simulink model "regulator_linear_2oder_T2"  (R2022b)
settings: Solver=VariableStepAuto  StartTime=0.0  StopTime=5  FixedStep=0.000001  RelTol=1e-3
values from neighbouring files (symbols this model uses):
  A = [0 1; -a0 -a1]    [analysis_effect_T.m]    (also in regulation_paramters.m)
  B = [b1; b0]    [analysis_effect_T.m]    (also in regulation_paramters.m)
  Pa = Popt    [analysis_effect_T.m]    (also in regulation_paramters.m)
  Q = eye(2)    [analysis_effect_T.m]    (also in regulation_paramters.m)
  R = 1    [analysis_effect_T.m]    (also in regulation_paramters.m)
  T2 = 0.005    [analysis_effect_T.m]
undefined symbols (not defined in the file or in its folder): Kopt, Popt
libraries: simulink x3, ctrlSharedLib x1
settings Model: Creator=acer  LastModifiedBy=dinhn

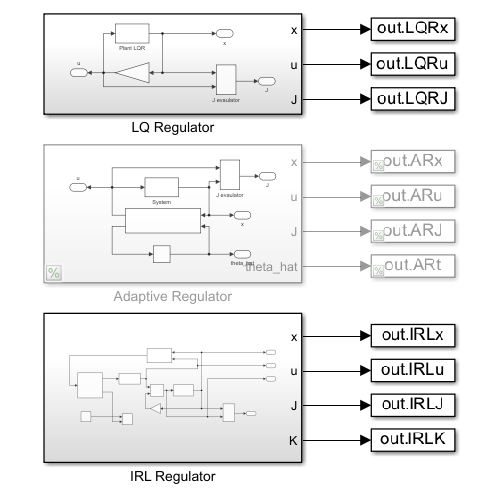
[thumbnail: Simulink's stored preview of the top-level diagram]
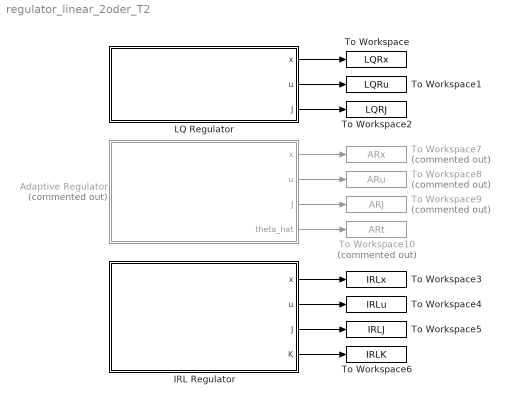
== system regulator_linear_2oder_T2 ==
  Adaptive Regulator : Subsystem  Commented=on
  IRL Regulator : Subsystem
  LQ Regulator : Subsystem
  To Workspace : ToWorkspace  VariableName=LQRx  SaveFormat=Timeseries  SampleTime=-1
  To Workspace1 : ToWorkspace  VariableName=LQRu  SaveFormat=Timeseries  SampleTime=-1
  To Workspace10 : ToWorkspace  Commented=on  VariableName=ARt  SaveFormat=Timeseries  SampleTime=-1
  To Workspace2 : ToWorkspace  VariableName=LQRJ  SaveFormat=Timeseries  SampleTime=-1
  To Workspace3 : ToWorkspace  VariableName=IRLx  SaveFormat=Timeseries  SampleTime=-1
  To Workspace4 : ToWorkspace  VariableName=IRLu  SaveFormat=Timeseries  SampleTime=-1
  To Workspace5 : ToWorkspace  VariableName=IRLJ  SaveFormat=Timeseries  SampleTime=-1
  To Workspace6 : ToWorkspace  VariableName=IRLK  SaveFormat=Timeseries  SampleTime=-1
  To Workspace7 : ToWorkspace  Commented=on  VariableName=ARx  SaveFormat=Timeseries  SampleTime=-1
  To Workspace8 : ToWorkspace  Commented=on  VariableName=ARu  SaveFormat=Timeseries  SampleTime=-1
  To Workspace9 : ToWorkspace  Commented=on  VariableName=ARJ  SaveFormat=Timeseries  SampleTime=-1
  wires:
  LQ Regulator/1(x) -> To Workspace/1
  LQ Regulator/2(u) -> To Workspace1/1
  LQ Regulator/3(J) -> To Workspace2/1
  Adaptive Regulator/1(x) -> To Workspace7/1
  Adaptive Regulator/2(u) -> To Workspace8/1
  Adaptive Regulator/3(J) -> To Workspace9/1
  Adaptive Regulator/4(theta_hat) -> To Workspace10/1
  IRL Regulator/1(x) -> To Workspace3/1
  IRL Regulator/2(u) -> To Workspace4/1
  IRL Regulator/3(J) -> To Workspace5/1
  IRL Regulator/4(K) -> To Workspace6/1

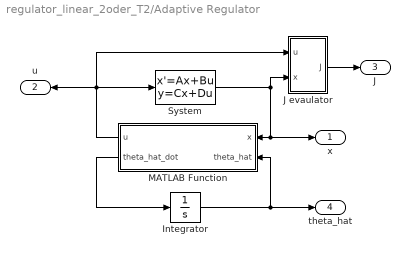
== system regulator_linear_2oder_T2/Adaptive Regulator ==
  Integrator : Integrator  InitialCondition=[0;0]
  J evaulator : Subsystem
  MATLAB Function : MATLAB Function  TreatAsAtomicUnit=on
  System : StateSpace  A=A  B=B  C=eye(2)  D=[0;0]  InitialCondition=[10;5]
  x : Outport
  u : Outport  Port=2
  J : Outport  Port=3
  theta_hat : Outport  Port=4
  wires:
  System/1 -> J evaulator/2(x), x/1, MATLAB Function/1(x)
  Integrator/1 -> theta_hat/1, MATLAB Function/2(theta_hat)
  MATLAB Function/2(theta_hat_dot) -> Integrator/1
  MATLAB Function/1(u) -> J evaulator/1(u), u/1, System/1
  J evaulator/1(J) -> J/1

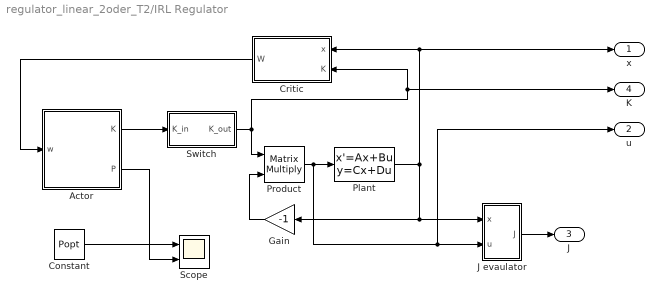
== system regulator_linear_2oder_T2/IRL Regulator ==
  Actor : MATLAB Function  TreatAsAtomicUnit=on
  Constant : Constant  Value=Popt
  Critic : Subsystem
  Gain : Gain  Gain=-1
  J evaulator : Subsystem
  Plant : StateSpace  A=A  B=B  C=eye(2)  D=[0;0]  InitialCondition=[10;5]  ParameterTunability=Unconstrained
  Product : Product  Multiplication=Matrix(*)
  Scope : Scope  NumInputPorts=2
  Switch : Subsystem
  x : Outport
  u : Outport  Port=2
  J : Outport  Port=3
  K : Outport  Port=4
  wires:
  Product/1 -> Plant/1, u/1, J evaulator/2(u)
  Constant/1 -> Scope/1
  Actor/2(P) -> Scope/2
  Critic/1(W) -> Actor/1(w)
  Actor/1(K) -> Switch/1(K_in)
  Switch/1(K_out) -> Critic/2(K), K/1, Product/1
  Plant/1 -> x/1, Critic/1(x), Gain/1, J evaulator/1(x)
  Gain/1 -> Product/2
  J evaulator/1(J) -> J/1

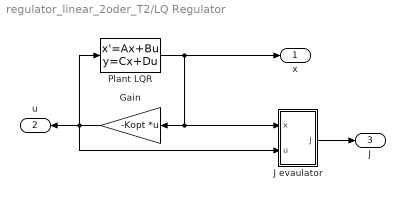
== system regulator_linear_2oder_T2/LQ Regulator ==
  Gain : Gain  Gain=-Kopt  Multiplication=Matrix(K*u)
  J evaulator : Subsystem
  Plant LQR : StateSpace  A=A  B=B  C=eye(2)  D=[0;0]  InitialCondition=[10;5]
  x : Outport
  u : Outport  Port=2
  J : Outport  Port=3
  wires:
  Gain/1 -> Plant LQR/1, u/1, J evaulator/2(u)
  Plant LQR/1 -> J evaulator/1(x), Gain/1, x/1
  J evaulator/1(J) -> J/1

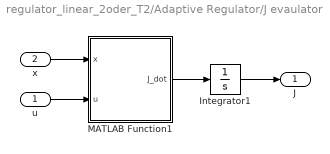
== system regulator_linear_2oder_T2/Adaptive Regulator/J evaulator ==
  u : Inport
  x : Inport  Port=2
  Integrator1 : Integrator
  MATLAB Function1 : MATLAB Function  TreatAsAtomicUnit=on
  J : Outport
  wires:
  Integrator1/1 -> J/1
  MATLAB Function1/1(J_dot) -> Integrator1/1
  x/1 -> MATLAB Function1/1(x)
  u/1 -> MATLAB Function1/2(u)

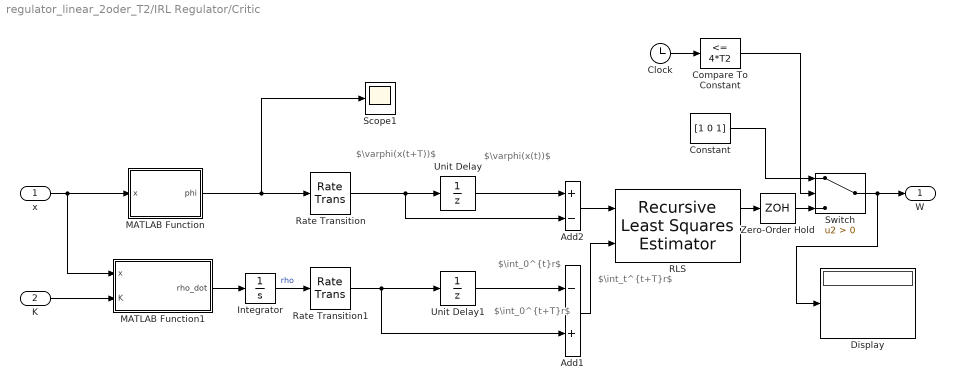
== system regulator_linear_2oder_T2/IRL Regulator/Critic ==
  note: $\varphi(x(t+T))$
  note: $\int_0^{t+T}r$
  note: $\int_t^{t+T}r$
  note: $\int_0^{t}r$
  note: $\varphi(x(t))$
  x : Inport
  K : Inport  Port=2
  Add1 : Sum  Inputs=-+
  Add2 : Sum  Inputs=+-
  Clock : Clock
  Compare To Constant : simulink/Logic and Bit Operations/Compare To Constant  relop=<=  const=4*T2  OutDataTypeStr=boolean
  Constant : Constant  Value=[1 0 1]
  Display : Display
  Integrator : Integrator
  MATLAB Function : MATLAB Function  TreatAsAtomicUnit=on
  MATLAB Function1 : MATLAB Function  TreatAsAtomicUnit=on
  RLS : ctrlSharedLib/Recursive Least Squares Estimator  InitialEstimateSource=Internal  InitialParameterData=[1 0 1]  P0=1  InitialRegressors=0  InitialOutputs=0  History=Finite  WindowLength=4  EstimationMethod=Forgetting Factor  AdaptationParameter=0  HasTimeVaryingAdaptationParameter=off  NormalizationBias=eps  OutputError=on  OutputP=off  AddEnablePort=off  InputProcessing=Sample-based  Ts=T2
  Rate Transition : RateTransition  InitialCondition=[100,60,9]  OutPortSampleTime=T2
  Rate Transition1 : RateTransition  OutPortSampleTime=T2
  Scope1 : Scope
  Switch : Switch  Criteria=u2 > Threshold  SaturateOnIntegerOverflow=off  InputSameDT=off
  Unit Delay : UnitDelay  InitialCondition=[100,60,9]  SampleTime=T2  HasFrameUpgradeWarning=on
  Unit Delay1 : UnitDelay  SampleTime=T2  HasFrameUpgradeWarning=on
  Zero-Order Hold : ZeroOrderHold  SampleTime=4*T2
  W : Outport
  wires:
  Add1/1 -> RLS/2
  Rate Transition/1 -> Add2/2, Unit Delay/1
  Rate Transition1/1 -> Add1/2, Unit Delay1/1
  Add2/1 -> RLS/1
  Unit Delay/1 -> Add2/1
  x/1 -> MATLAB Function1/1(x), MATLAB Function/1(x)
  MATLAB Function1/1(rho_dot) -> Integrator/1
  Unit Delay1/1 -> Add1/1
  Integrator/1 -> Rate Transition1/1  "rho"
  MATLAB Function/1(phi) -> Scope1/1, Rate Transition/1
  K/1 -> MATLAB Function1/2(K)
  RLS/1 -> Zero-Order Hold/1
  Clock/1 -> Compare To Constant/1
  Compare To Constant/1 -> Switch/2
  Constant/1 -> Switch/1
  Switch/1 -> Display/1, W/1
  Zero-Order Hold/1 -> Switch/3

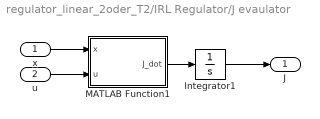
== system regulator_linear_2oder_T2/IRL Regulator/J evaulator ==
  x : Inport
  u : Inport  Port=2
  Integrator1 : Integrator
  MATLAB Function1 : MATLAB Function  TreatAsAtomicUnit=on
  J : Outport
  wires:
  Integrator1/1 -> J/1
  MATLAB Function1/1(J_dot) -> Integrator1/1
  x/1 -> MATLAB Function1/1(x)
  u/1 -> MATLAB Function1/2(u)

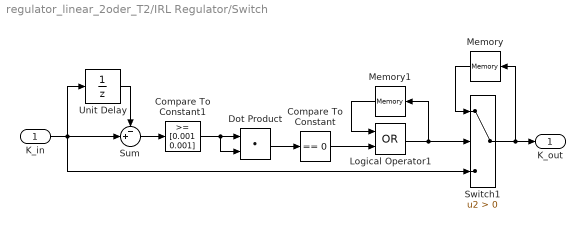
== system regulator_linear_2oder_T2/IRL Regulator/Switch ==
  K_in : Inport
  Compare To Constant : simulink/Logic and Bit Operations/Compare To Constant  relop===  const=0  OutDataTypeStr=boolean
  Compare To Constant1 : simulink/Logic and Bit Operations/Compare To Constant  relop=>=  const=[0.001 0.001]  OutDataTypeStr=boolean
  Dot Product : DotProduct  OutDataTypeStr=Inherit: Inherit via internal rule
  Logical Operator1 : Logic  Operator=OR  AllPortsSameDT=off  OutDataTypeStr=boolean
  Memory : Memory
  Memory1 : Memory
  Sum : Sum  Inputs=-+|
  Switch1 : Switch  Criteria=u2 > Threshold  SaturateOnIntegerOverflow=off  InputSameDT=off
  Unit Delay : UnitDelay  SampleTime=3*4*T2  HasFrameUpgradeWarning=on
  K_out : Outport
  wires:
  K_in/1 -> Sum/2, Unit Delay/1, Switch1/3
  Switch1/1 -> K_out/1, Memory/1
  Compare To Constant1/1 -> Dot Product/2, Dot Product/1
  Sum/1 -> Compare To Constant1/1
  Dot Product/1 -> Compare To Constant/1
  Memory/1 -> Switch1/1
  Logical Operator1/1 -> Memory1/1, Switch1/2
  Compare To Constant/1 -> Logical Operator1/2
  Memory1/1 -> Logical Operator1/1
  Unit Delay/1 -> Sum/1

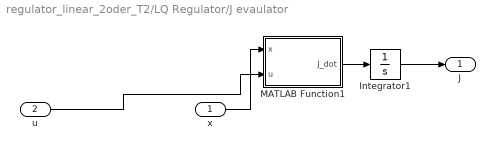
== system regulator_linear_2oder_T2/LQ Regulator/J evaulator ==
  x : Inport
  u : Inport  Port=2
  Integrator1 : Integrator
  MATLAB Function1 : MATLAB Function  TreatAsAtomicUnit=on
  J : Outport
  wires:
  Integrator1/1 -> J/1
  MATLAB Function1/1(J_dot) -> Integrator1/1
  x/1 -> MATLAB Function1/1(x)
  u/1 -> MATLAB Function1/2(u)

== matlab function regulator_linear_2oder_T2/IRL Regulator/Actor ==
  data: K output; w input; R parameter; B parameter; P output
function [K, P] = fcn(w, R, B)

P = [w(1), w(2);
     w(2), w(3)];

K = R \ B' * P;

== matlab function regulator_linear_2oder_T2/IRL Regulator/Critic/MATLAB Function ==
  data: x input; phi output
function phi = fcn(x)

phi11 = x(1)*x(1);
phi12 = x(1)*x(2);
phi22 = x(2)*x(2);

phi = [phi11 2*phi12 phi22];

== matlab function regulator_linear_2oder_T2/IRL Regulator/Critic/MATLAB Function1 ==
  data: x input; rho_dot output; K input; R parameter; Q parameter
function rho_dot = fcn(x, K, R, Q)

rho_dot = x' * (Q + K' * R * K) * x;

== matlab function regulator_linear_2oder_T2/IRL Regulator/J evaulator/MATLAB Function1 ==
  data: x input; u input; J_dot output; Q parameter; R parameter
function J_dot = fcn(x,u,Q,R)

J_dot = x' * Q * x + u' * R * u;

== matlab function regulator_linear_2oder_T2/LQ Regulator/J evaulator/MATLAB Function1 ==
  data: x input; u input; J_dot output; Q parameter; R parameter
function J_dot = fcn(x,u,Q,R)

J_dot = x' * Q * x + u' * R * u;

== matlab function regulator_linear_2oder_T2/Adaptive Regulator/MATLAB Function ==
  data: x input; u output; theta_hat input; theta_hat_dot output; B parameter; Pa parameter
function [u, theta_hat_dot] = fcn(x,theta_hat,B, Pa)
gamma = 1;
theta_hat_dot = gamma * x * B' * Pa * x;
u = -theta_hat' * x;

== matlab function regulator_linear_2oder_T2/Adaptive Regulator/J evaulator/MATLAB Function1 ==
  data: x input; u input; J_dot output; Q parameter; R parameter
function J_dot = fcn(x,u,Q,R)

J_dot = x' * Q * x + u' * R * u;
